simulink library "Regulators_library"  (R2023b)
settings: Solver=VariableStepAuto  StartTime=0.0  StopTime=10.0  RelTol=1e-3
libraries: simulink x1
settings Model: Creator=Student  LastModifiedBy=Student

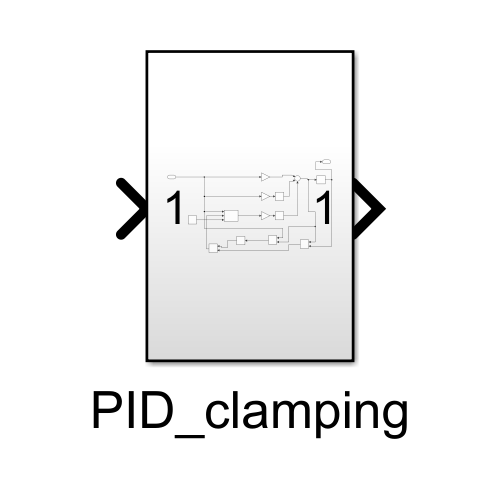
[thumbnail: Simulink's stored preview of the top-level diagram]
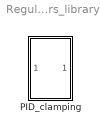
== system Regulators_library ==
  PID_clamping : Subsystem

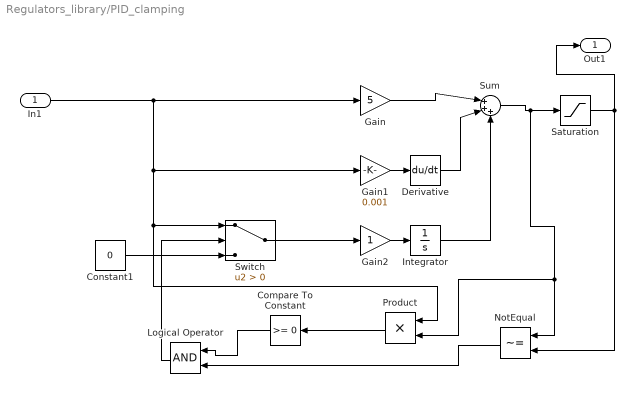
== system Regulators_library/PID_clamping ==
  In1 : Inport
  Compare To Constant : simulink/Logic and Bit Operations/Compare To Constant  relop=>=  const=0  OutDataTypeStr=boolean
  Constant1 : Constant  Value=0
  Derivative : Derivative
  Gain : Gain  Gain=5
  Gain1 : Gain  Gain=0.001
  Gain2 : Gain
  Integrator : Integrator
  Logical Operator : Logic  AllPortsSameDT=off  OutDataTypeStr=boolean
  NotEqual : RelationalOperator  Operator=~=  OutDataTypeStr=boolean  RndMeth=Simplest  InputSameDT=off
  Product : Product
  Saturation : Saturate  UpperLimit=30  LowerLimit=-250
  Sum : Sum  Inputs=|+++
  Switch : Switch  Criteria=u2 > Threshold  SaturateOnIntegerOverflow=off  InputSameDT=off
  Out1 : Outport
  wires:
  Derivative/1 -> Sum/2
  Gain2/1 -> Integrator/1
  Switch/1 -> Gain2/1
  Sum/1 -> Product/2, NotEqual/1, Saturation/1
  Gain1/1 -> Derivative/1
  Integrator/1 -> Sum/3
  Saturation/1 -> Out1/1, NotEqual/2
  Logical Operator/1 -> Switch/2
  In1/1 -> Switch/1, Product/1, Gain1/1, Gain/1
  Product/1 -> Compare To Constant/1
  NotEqual/1 -> Logical Operator/2
  Compare To Constant/1 -> Logical Operator/1
  Constant1/1 -> Switch/3
  Gain/1 -> Sum/1
